simulink model "admittance_controller_transl"  (R2021b)
settings: Solver=VariableStepAuto  StartTime=0.0  StopTime=10.0  RelTol=1e-3
undefined symbols (not defined in the file): ddp_d, dp_d, f, p_d
settings Model: Creator=Martin  LastModifiedBy=Martin

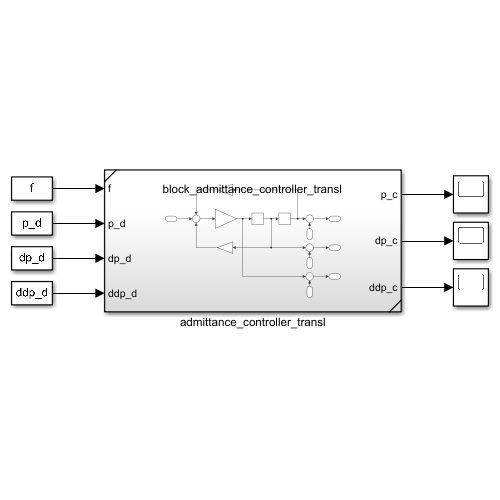
[thumbnail: Simulink's stored preview of the top-level diagram]
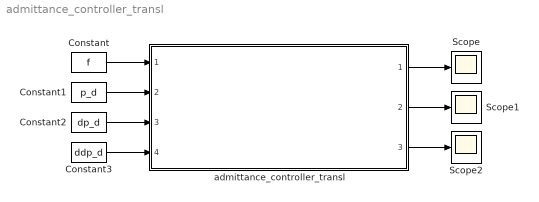
== system admittance_controller_transl ==
  Constant : Constant  Value=f  VectorParams1D=off
  Constant1 : Constant  Value=p_d  VectorParams1D=off
  Constant2 : Constant  Value=dp_d  VectorParams1D=off
  Constant3 : Constant  Value=ddp_d  VectorParams1D=off
  Scope : Scope
  Scope1 : Scope
  Scope2 : Scope
  admittance_controller_transl : Subsystem  ReferencedSubsystem=block_admittance_controller_transl
  wires:
  Constant/1 -> admittance_controller_transl/1
  Constant1/1 -> admittance_controller_transl/2
  Constant2/1 -> admittance_controller_transl/3
  Constant3/1 -> admittance_controller_transl/4
  admittance_controller_transl/1 -> Scope/1
  admittance_controller_transl/2 -> Scope1/1
  admittance_controller_transl/3 -> Scope2/1
